simulink library "commcrc2"  (Simulink 6.0)
settings: Solver=ode45  SolverMode=SingleTasking  StartTime=0.0  StopTime=10.0  RelTol=1e-3
libraries: commcrc2 x2
settings Model: Creator=akansal  LastModifiedBy=cvora  ExtModeAutoUpdateStatusClock=off
settings DataIOCC: SignalLoggingName=logsOut
settings OptimizationCC: BooleanDataType=off
settings DebuggingCC: CheckExecutionContextPreStartOutputMsg=on  CheckExecutionContextRuntimeOutputMsg=on  SolverPrmCheckMsg=none
settings HardwareCC: TargetUnknown=on
settings SFSimCC: SFSimApplyToAllLibs=on  SFSimBuildMode=Incremental

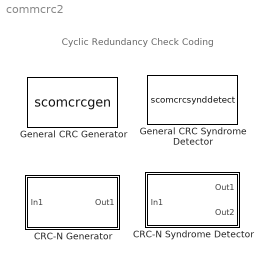
== system commcrc2 ==
  note: Cyclic Redundancy Check Coding
  CRC-N Generator : Subsystem  PropExecContextAcrossSSBoundary=on  mask(CRC-N Generator){crcMethod=CRC-16, iniStates=[0], numChecksums=1}
      mask prompts: crcMethod "CRC method:"; iniStates "Initial States:"; numChecksums "Checksums per frame:"
      mask help:
      | Generate CRC bits according to the selected CRC method and append them to the input data frames. The CRC method uses a pre-defined CRC-N polynomial where N is the number of bits in the checksum.
      |
      | The initial states parameter must be a binary scalar or vector of length equal to N.
      |
      | The input must be a binary frame-based column vector.
      mask init:
      | if strcmp(crcMethod, 'CRC-32')
      |    genPoly = [1 0 0 0 0 0 1 0 0 1 1 0 0 0 0 0 1 0 0 0 1 1 1 0 1 1 0 1 1 0 1 1 1];
      | elseif strcmp(crcMethod, 'CRC-24')
      |    genPoly = [1 1 0 0 0 0 0 0 0 0 1 0 1 0 0 0 1 0 0 0 0 0 0 0 1];
      | elseif strcmp(crcMethod, 'CRC-16')
      |    genPoly = [1 1 0 0 0 0 0 0 0 0 0 0 0 0 1 0 1];
      | elseif strcmp(crcMethod, 'Reversed CRC-16')
      |    genPoly = [1 0 1 0 0 0 0 0 0 0 0 0 0 0 0 1 1];
      | elseif strcmp(crcMethod, 'CRC-8')
      |    genPoly = [1 1 1 0 1 0 1 0 1];
      | elseif strcmp(crcMethod, 'CRC-4')
      |    genPoly = [1 1 1 1 1];
      | end
      mask Help: helpview(commbhelp);
      mask StyleString: popup(CRC-32|CRC-24|CRC-16|Reversed CRC-16|CRC-8|CRC-4),edit,edit
      mask Display: disp('CRC-N\nGenerator');
  CRC-N Syndrome Detector : Subsystem  PropExecContextAcrossSSBoundary=on  mask(CRC-N Syndrome Detector){crcMethod=CRC-16, iniStates=[0], numChecksums=1}
      mask prompts: crcMethod "CRC method:"; iniStates "Initial states:"; numChecksums "Checksums per frame:"
      mask help:
      | Detect errors in the input data frames according to the selected CRC method. The CRC method uses a pre-defined CRC-N polynomial where N is the number of bits in the checksum.
      |
      | The first output is the data frame with the CRC bits removed and the second output indicates if an error was detected in the data frame.
      |
      | The initial states parameter must be a binary scalar or vector of length equal to N.
      |
      | The input must be a binary frame-based column vector.
      mask init: same as commcrc2/CRC-N Generator
      mask Help: helpview(commbhelp);
      mask StyleString: popup(CRC-32|CRC-24|CRC-16|Reversed CRC-16|CRC-8|CRC-4),edit,edit
      mask Display:
      | disp('CRC-N\nSyndrome\nDetector');
      | port_label('output',2,'Err');
  General CRC Generator : S-Function  FunctionName=scomcrcgen  Parameters=genPoly, numBits, iniStates, numChecksums  mask(General CRC Generator){genPoly=[1 0 0 0 1 0 0 0 0 0 0 1 0 0 0 0 1], iniStates=[0], numChecksums=1}
      mask prompts: genPoly "Generator polynomial:"; iniStates "Initial states:"; numChecksums "Checksums per frame:"
      mask help:
      | Generate CRC bits according to the generator polynomial and append them to the input data frames. The generator polynomial must be specified as a binary vector or a descending ordered polynomial, to indicate the connection points.
      |
      | The initial states parameter must be a binary scalar or vector of length equal to the degree of the polynomial.
      |
      | The input must be a binary frame-based column vector.
      mask init:
      | [genPoly, numBits, iniStates, numChecksums] = commblkcrcgen(genPoly, iniStates, numChecksums);
      mask Help: helpview(commbhelp);
      mask Display: disp('General\nCRC\nGenerator');
  General CRC Syndrome Detector : S-Function  FunctionName=scomcrcsynddetect  Parameters=genPoly, numBits, iniStates, numChecksums  mask(General CRC Syndrome Detector){genPoly=[1 0 0 0 1 0 0 0 0 0 0 1 0 0 0 0 1], iniStates=[0], numChecksums=1}
      mask prompts: genPoly "Generator polynomial:"; iniStates "Initial states:"; numChecksums "Checksums per frame:"
      mask help:
      | Detect errors in the input data frames according to the generator polynomial. The generator polynomial must be specified as a binary vector or a descending ordered polynomial, to indicate the connection points.
      |
      | The first output is the data frame with the CRC bits removed and the second output indicates if an error was detected in the data frame.
      |
      | The initial states parameter must be a binary scalar or vector of length equal to the degree of the polynomial.
      |
      | The input must be a binary frame-based column vector.
      mask init:
      | [genPoly, numBits, iniStates, numChecksums] = commblkcrcgen(genPoly, iniStates, numChecksums);
      mask Help: helpview(commbhelp);
      mask Display:
      | disp('General CRC\nSyndrome\nDetector');
      | port_label('output',2,'Err');

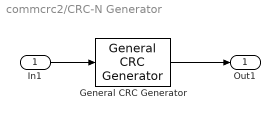
== system commcrc2/CRC-N Generator ==
  In1 : Inport  LatchInput=off
  General CRC Generator : commcrc2/General CRC Generator  genPoly=genPoly  iniStates=iniStates  numChecksums=numChecksums
  Out1 : Outport
  wires:
  In1/1 -> General CRC Generator/1
  General CRC Generator/1 -> Out1/1

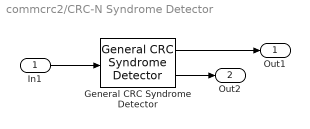
== system commcrc2/CRC-N Syndrome Detector ==
  In1 : Inport  LatchInput=off
  General CRC Syndrome Detector : commcrc2/General CRC Syndrome Detector  genPoly=genPoly  iniStates=iniStates  numChecksums=numChecksums
  Out1 : Outport
  Out2 : Outport  Port=2
  wires:
  General CRC Syndrome Detector/2 -> Out2/1
  General CRC Syndrome Detector/1 -> Out1/1
  In1/1 -> General CRC Syndrome Detector/1
